simulink model "SFcontroleur5"  (R2020a)
settings: Solver=VariableStepAuto  StartTime=0.0  StopTime=inf  RelTol=1e-3
settings Model: Creator=maxen  LastModifiedBy=maxen

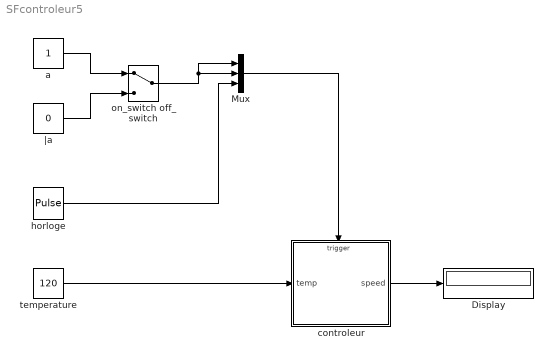
== system SFcontroleur5 ==
  Display : Display
  Mux : Mux  Inputs=3
  a : Constant
  controleur : Stateflow chart  TreatAsAtomicUnit=on
  horloge : DiscretePulseGenerator  PulseType=Time based  Period=1  PulseWidth=5
  on_switch off_switch : ManualSwitch
  temperature : Constant  Value=120
  |a : Constant  Value=0
  wires:
  |a/1 -> on_switch off_switch/2
  a/1 -> on_switch off_switch/1
  on_switch off_switch/1 -> Mux/2, Mux/1
  Mux/1 -> controleur/Trigger
  controleur/1(speed) -> Display/1
  horloge/1 -> Mux/3
  temperature/1 -> controleur/1(temp)

== stateflow chart SFcontroleur5/controleur ==
  settings: executeAtInitialization=1
  state On
    (history)
    state High
      en:speed = 2;
    state Low
      en:speed = 1;
    Low -> High : [hot()]
    High -> Low : [~hot()]
    (default) -> Low
  state Off
    en:speed = 0;
  state r=hot [function]
    (default) -> (junction 54) : {r=temp>=120;}
  Off -> On : on_switch
  On -> Off : off_switch
  (default) -> Off
  data: r function_output; speed output; temp input
  events: off_switch input FALLING_EDGE_EVENT; on_switch input RISING_EDGE_EVENT; temp_event input RISING_EDGE_EVENT
